simulink model "sfunction"  (R2019a)
settings: Solver=ode45  StartTime=0.0  StopTime=10.0  RelTol=1e-3
settings Model: Creator=24249  LastModifiedBy=24249

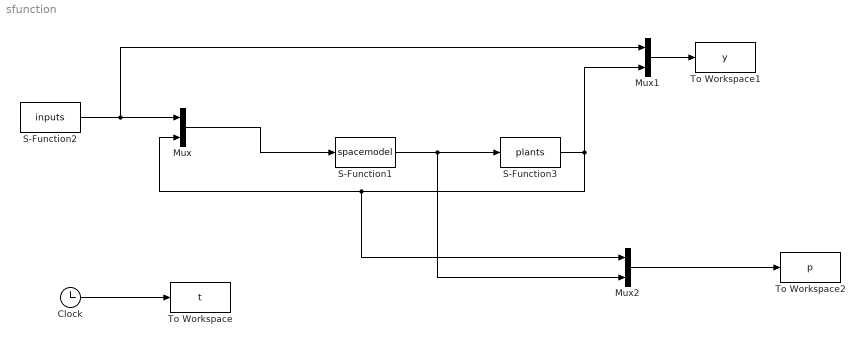
== system sfunction ==
  Clock : Clock
  Mux : Mux  Inputs=2
  Mux1 : Mux  Inputs=2
  Mux2 : Mux  Inputs=2
  S-Function1 : S-Function  FunctionName=spacemodel  SFunctionDeploymentMode=off  EnableBusSupport=off
  S-Function2 : S-Function  FunctionName=inputs  SFunctionDeploymentMode=off  EnableBusSupport=off
  S-Function3 : S-Function  FunctionName=plants  SFunctionDeploymentMode=off  EnableBusSupport=off
  To Workspace : ToWorkspace  VariableName=t  SaveFormat=Structure With Time  SampleTime=-1
  To Workspace1 : ToWorkspace  VariableName=y  SaveFormat=Structure With Time  SampleTime=-1
  To Workspace2 : ToWorkspace  VariableName=p  SaveFormat=Structure With Time  SampleTime=-1
  wires:
  Clock/1 -> To Workspace/1
  S-Function1/1 -> Mux2/2, S-Function3/1
  S-Function2/1 -> Mux1/1, Mux/1
  S-Function3/1 -> Mux1/2, Mux2/1, Mux/2
  Mux/1 -> S-Function1/1
  Mux1/1 -> To Workspace1/1
  Mux2/1 -> To Workspace2/1
